simulink model "fivelevels"  (R2017b)
settings: Solver=VariableStepAuto  StartTime=0.0  StopTime=10.0  MaxStep=1e-4  RelTol=1e-3
libraries: powerlib x13
settings Model: Creator=Admin  LastModifiedBy=Admin

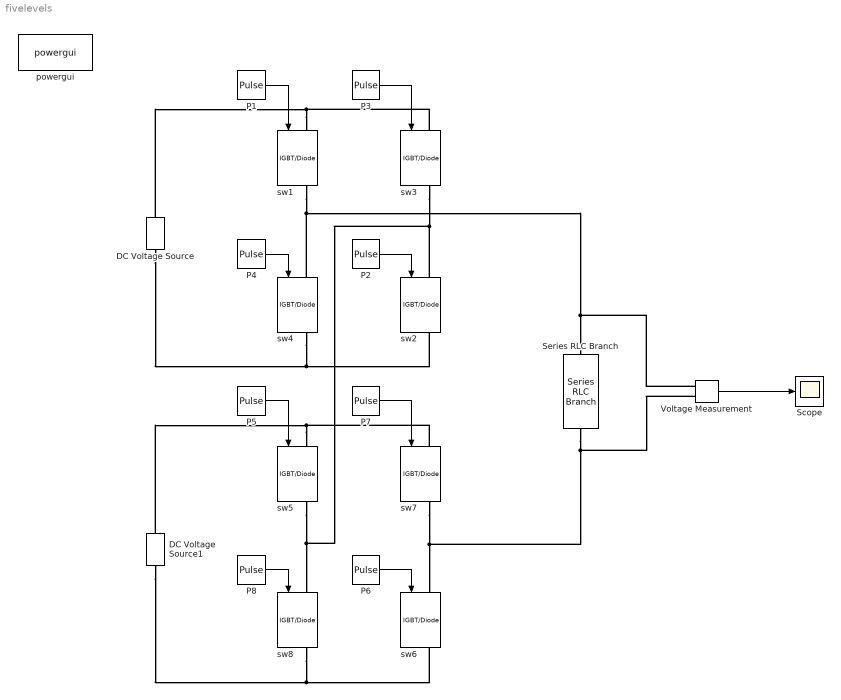
== system fivelevels ==
  DC Voltage Source : powerlib/Electrical Sources/DC Voltage Source  Amplitude=100  Measurements=None
  DC Voltage Source1 : powerlib/Electrical Sources/DC Voltage Source  Amplitude=100  Measurements=None
  P1 : DiscretePulseGenerator  PulseType=Time based  Period=0.02  PulseWidth=30  PhaseDelay=0.002
  P2 : DiscretePulseGenerator  PulseType=Time based  Period=0.02  PulseWidth=30  PhaseDelay=0.002
  P3 : DiscretePulseGenerator  PulseType=Time based  Period=0.02  PulseWidth=10  PhaseDelay=0.014
  P4 : DiscretePulseGenerator  PulseType=Time based  Period=0.02  PulseWidth=30  PhaseDelay=0.012
  P5 : DiscretePulseGenerator  PulseType=Time based  Period=0.02  PulseWidth=10  PhaseDelay=0.004
  P6 : DiscretePulseGenerator  PulseType=Time based  Period=0.02  PulseWidth=30  PhaseDelay=0.002
  P7 : DiscretePulseGenerator  PulseType=Time based  Period=0.02  PulseWidth=30  PhaseDelay=0.012
  P8 : DiscretePulseGenerator  PulseType=Time based  Period=0.02  PulseWidth=30  PhaseDelay=0.012
  Scope : Scope
  Series RLC Branch : powerlib/Elements/Series RLC Branch  LConnTagsString=__new0  RConnTagsString=__new0  BranchType=R  Resistance=1  Inductance=1e-3  SetiL0=off  InitialCurrent=0  Capacitance=1e-6  Setx0=off  InitialVoltage=0  Measurements=None
  Voltage Measurement : powerlib/Measurements/Voltage Measurement  PhasorSimulation=off  OutputType=Complex  PSBequivalent=0
  powergui : powerlib/powergui  Priority=1  SimulationMode=Continuous  SampleTime=50e-6  frequency=60  Iterations=50  frequencyindice=0  Pbase=100e6  ErrMax=1e-4  UnitsV=kV  UnitsW=MW  buscounter=0  FunctionMessages=off  echomessages=off  EnableUseOfTLC=off  CurrentSourceSwitches=off  DisableSnubberDevices=off  DisableRonSwitches=off  DisableVfSwitches=off  DisplayEquations=off  SolverType=Tustin/Backward Euler (TBE)  Interpol=off  ExternalGateDelay=off  methode=off  Ts=100  x0status=blocks  SPID=on  SwTol=0  HookPort=off  RestoreLinks=warning  ResistiveCurrentMeasurement=off  Frange=[0:2:500]  Ylog=off  Xlog=on  ShowGrid=off  save=off  variable=ZData  structure=0  ZoomFFT=off  StartTime=0.0  cycles=1  DisplayStyle=1  fundamental=60  FreqAxis=off  MaxFrequency=1000  frequencyindicesteady=1  RmsSteady=1  display=off
  sw{1..3,5..8} (7 alike) : powerlib/Power Electronics/IGBT//Diode  Ron=1e-3  Rs=1e5  Cs=inf  Measurements=on
  "sw4 " : powerlib/Power Electronics/IGBT//Diode  Ron=1e-3  Rs=1e5  Cs=inf  Measurements=on
  wires:
  Voltage Measurement/1 -> Scope/1
  P1/1 -> sw1/1
  P4/1 -> "sw4 "/1
  P2/1 -> sw2/1
  P3/1 -> sw3/1
  P5/1 -> sw5/1
  P8/1 -> sw8/1
  P6/1 -> sw6/1
  P7/1 -> sw7/1
  connections:
  sw1/LConn1 -- sw3/LConn1 -- DC Voltage Source/RConn1
  sw2/RConn1 -- "sw4 "/RConn1 -- DC Voltage Source/LConn1
  sw5/LConn1 -- sw7/LConn1 -- DC Voltage Source1/RConn1
  sw6/RConn1 -- sw8/RConn1 -- DC Voltage Source1/LConn1
  sw7/RConn1 -- Voltage Measurement/LConn2 -- Series RLC Branch/RConn1 -- sw6/LConn1
  sw1/RConn1 -- "sw4 "/LConn1 -- Voltage Measurement/LConn1 -- Series RLC Branch/LConn1
  sw5/RConn1 -- sw3/RConn1 -- sw2/LConn1 -- sw8/LConn1
